simulink model "THREE_LEVEL_INV"  (R2015a)
settings: Solver=ode3  StartTime=0.0  StopTime=10.0  RelTol=1e-3
libraries: powerlib x9, arduinolib x5
settings Model: ExtModeTrigDuration=2  Creator=Anand  LastModifiedBy=AKGC
settings OptimizationCC: OptimizeModelRefInitCode=on  LifeSpan=1
settings DebuggingCC: UnderspecifiedInitializationDetection=Classic  MergeDetectMultiDrivingBlocksExec=none
settings HardwareCC: ProdBitPerInt=16  ProdBitPerPointer=8  ProdIntDivRoundTo=Zero  ProdEndianess=LittleEndian  ProdWordSize=8  ProdHWDeviceType=Atmel->AVR
settings RTWCC: SystemTargetFile=realtime.tlc  GenerateMakefile=off  TemplateMakefile=realtime.tmf  Description=Run on Target Hardware  RTWVerbose=off
settings ERTTargetCC: CombineOutputUpdateFcns=off  ExtModeTransport=3  ExtModeMexFile=ext_serial_win32_comm_rtt  ExtModeMexArgs=0 1 9600  ERTSrcFileBannerTemplate=realtime_code_template.cgt  ERTHdrFileBannerTemplate=realtime_code_template.cgt  ERTDataSrcFileTemplate=realtime_code_template.cgt  ERTDataHdrFileTemplate=realtime_code_template.cgt  ERTCustomFileTemplate=realtime_file_process.tlc

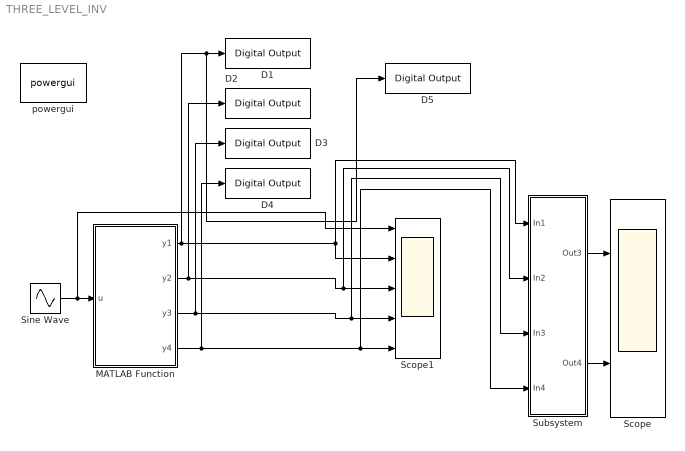
== system THREE_LEVEL_INV ==
  D1 : arduinolib/Digital Output  pinNumber=22  blockPlatform=arduino
  D2 : arduinolib/Digital Output  pinNumber=23  blockPlatform=arduino
  D3 : arduinolib/Digital Output  pinNumber=24  blockPlatform=arduino
  D4 : arduinolib/Digital Output  pinNumber=25  blockPlatform=arduino
  D5 : arduinolib/Digital Output  pinNumber=13  blockPlatform=arduino
  MATLAB Function : MATLAB Function  TreatAsAtomicUnit=on
  Scope : Scope  NumInputPorts=2
      settings: YMin=-5~-5  YMax=5~5
  Scope1 : Scope  NumInputPorts=5
      settings: YMin=-5~-5~-5~-5~-5  YMax=5~5~5~5~5
  Sine Wave : Sin  Amplitude=5  Frequency=314.159265  SampleTime=0.00055555
  Subsystem : Subsystem
  powergui : powerlib/powergui  Priority=1  SimulationMode=Continuous  SolverType=Tustin/Backward Euler (TBE)  SampleTime=50e-6  frequency=60  SPID=off  DisableSnubberDevices=off  DisableRonSwitches=off  DisableVfSwitches=off  SwTol=0  DisplayEquations=off  Interpol=off  methode=off  Ts=100  FunctionMessages=off  echomessages=off  HookPort=off  EnableUseOfTLC=off  x0status=blocks  frequencyindice=0  Pbase=100e6  ErrMax=1e-4  Iterations=50  UnitsV=kV  UnitsW=MW  buscounter=0  RestoreLinks=warning  ResistiveCurrentMeasurement=off  Frange=[0:2:500]  Ylog=off  Xlog=on  ShowGrid=off  save=off  variable=ZData  structure=0  ZoomFFT=off  StartTime=0.0  cycles=1  DisplayStyle=1  fundamental=60  FreqAxis=off  MaxFrequency=1000  frequencyindicesteady=1  RmsSteady=1  display=off
  wires:
  Sine Wave/1 -> Scope1/1, MATLAB Function/1(u)
  MATLAB Function/1(y1) -> D5/1, D1/1, Scope1/2, Subsystem/1(In1)
  MATLAB Function/2(y2) -> D2/1, Subsystem/2(In2), Scope1/3
  MATLAB Function/3(y3) -> D3/1, Scope1/4, Subsystem/3(In3)
  MATLAB Function/4(y4) -> D4/1, Scope1/5, Subsystem/4(In4)
  Subsystem/1(Out3) -> Scope/1
  Subsystem/2(Out4) -> Scope/2

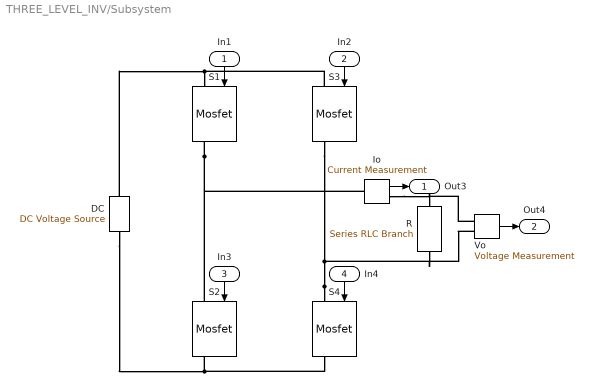
== system THREE_LEVEL_INV/Subsystem ==
  In1 : Inport
  In2 : Inport  Port=2
  In3 : Inport  Port=3
  In4 : Inport  Port=4
  "DC " : powerlib/Electrical Sources/DC Voltage Source  Amplitude=100  Measurements=None
  Io : powerlib/Measurements/Current Measurement  PhasorSimulation=off  OutputType=Complex  PSBequivalent=0
  R : powerlib/Elements/Series RLC Branch  LConnTagsString=__new0  RConnTagsString=__new0  BranchType=R  Resistance=10  Inductance=1e-3  SetiL0=off  InitialCurrent=0  Capacitance=1e-6  Setx0=off  InitialVoltage=0  Measurements=None
  S{1..4} (4 alike) : powerlib/Power Electronics/Mosfet  Ron=0.1  Lon=0  Rd=0.01  Vfd=0  IC=0  Rs=1e5  Cs=inf  Measurements=on
  Vo : powerlib/Measurements/Voltage Measurement  PhasorSimulation=off  OutputType=Complex  PSBequivalent=0
  Out3 : Outport
  Out4 : Outport  Port=2
  wires:
  In3/1 -> S2/1
  Vo/1 -> Out4/1
  In2/1 -> S3/1
  In4/1 -> S4/1
  In1/1 -> S1/1
  Io/1 -> Out3/1
  connections:
  S2/RConn1 -- S4/RConn1 -- "DC "/LConn1
  S1/RConn1 -- S2/LConn1 -- Io/LConn1
  R/LConn1 -- Io/RConn1 -- Vo/LConn1
  S4/LConn1 -- S3/RConn1 -- Vo/LConn2 -- R/RConn1
  S1/LConn1 -- "DC "/RConn1 -- S3/LConn1

== matlab function THREE_LEVEL_INV/MATLAB Function ==
  data: u input; y1 output; y2 output; y3 output; y4 output
function [y1,y2,y3,y4] = fcn(u)

%Positive Cycle
        if(u>=0 && u<=1)
            y1=0; y2=0;y3=0; y4=0;      %Vo=0
        elseif(u>=1 && u<=9)
            y1=1; y2=0;y3=0; y4=1;      %Vo=+V1
        elseif(u>=9 && u<=10)
             y1=0; y2=0;y3=0; y4=0;     %Vo=0
 %Negative Cycle
        elseif(u<=-0 && u>=-1)
            y1=0; y2=0;y3=0; y4=0;      %Vo=0
        elseif(u<=-1 && u>=-9)
            y1=0; y2=1;y3=1; y4=0;      %Vo=+V1
        elseif(u<=-9 && u>=-10)
             y1=0; y2=0;y3=0; y4=0;     %Vo=0
        else
           y1=0; y2=0;y3=0; y4=0;      %Vo=0
        end
